simulink model "InjVlv_BlkSht"  (R2016b)
settings: configuration reference "CodeGenConfigSet" (kept outside this file)
values from neighbouring files (symbols this model uses):
  InjVlv_freqBlkShtMax_CUR = Calibration.Parameter    [init_InjVlv_BlkSht.m]    (also in init_InjVlv_BlkSht_SIL.m = Simulink.Parameter)
  InjVlv_freqBlkShtMax_CURX = Calibration.Parameter    [init_InjVlv_BlkSht.m]    (also in init_InjVlv_BlkSht_SIL.m = Simulink.Parameter)
  InjVlv_freqBlkShtMin_C = Calibration.Parameter    [init_InjVlv_BlkSht.m]    (also in init_InjVlv_BlkSht_SIL.m = Simulink.Parameter)
  InjVlv_phiBlkShtStrt_C = Calibration.Parameter    [init_InjVlv_BlkSht.m]    (also in init_InjVlv_BlkSht_SIL.m = Simulink.Parameter)
  InjVlv_phiBlkShtStrtMax_C = Calibration.Parameter    [init_InjVlv_BlkSht.m]    (also in init_InjVlv_BlkSht_SIL.m = Simulink.Parameter)
  InjVlv_phiBlkShtStrtMin_C = Calibration.Parameter    [init_InjVlv_BlkSht.m]    (also in init_InjVlv_BlkSht_SIL.m = Simulink.Parameter)
  InjVlv_swtPlausBlkShtET_C = Calibration.Parameter    [init_InjVlv_BlkSht.m]    (also in init_InjVlv_BlkSht_SIL.m = Simulink.Parameter)
  InjVlv_tiETBlkSht_MAP = Calibration.Parameter    [init_InjVlv_BlkSht.m]    (also in init_InjVlv_BlkSht_SIL.m = Simulink.Parameter)
  InjVlv_tiETBlkSht_MAPX = Calibration.Parameter    [init_InjVlv_BlkSht.m]    (also in init_InjVlv_BlkSht_SIL.m = Simulink.Parameter)
  InjVlv_tiETBlkSht_MAPY = Calibration.Parameter    [init_InjVlv_BlkSht.m]    (also in init_InjVlv_BlkSht_SIL.m = Simulink.Parameter)
  InjVlv_tiETBlkShtAft_MAP = Calibration.Parameter    [init_InjVlv_BlkSht.m]    (also in init_InjVlv_BlkSht_SIL.m = Simulink.Parameter)
  InjVlv_tiETBlkShtAft_MAPX = Calibration.Parameter    [init_InjVlv_BlkSht.m]    (also in init_InjVlv_BlkSht_SIL.m = Simulink.Parameter)
  InjVlv_tiETBlkShtAft_MAPY = Calibration.Parameter    [init_InjVlv_BlkSht.m]    (also in init_InjVlv_BlkSht_SIL.m = Simulink.Parameter)
  InjVlv_tiETBlkShtMin_C = Calibration.Parameter    [init_InjVlv_BlkSht.m]    (also in init_InjVlv_BlkSht_SIL.m = Simulink.Parameter)
  InjVlv_tiETBlkShtZFC_C = Calibration.Parameter    [init_InjVlv_BlkSht.m]    (also in init_InjVlv_BlkSht_SIL.m = Simulink.Parameter)
  SigTst_freqBlkSht_C = Calibration.Parameter    [init_InjVlv_BlkSht.m]    (also in init_InjVlv_BlkSht_SIL.m = Simulink.Parameter)
  SigTst_swtFreqBlkSht_C = Calibration.Parameter    [init_InjVlv_BlkSht.m]    (also in init_InjVlv_BlkSht_SIL.m = Simulink.Parameter)
undefined symbols (not defined in the file or in its folder): Rail_BlkShtMode_VERB, SubSysExeState_conv, Switch_conv
libraries: CXLib x1
settings Model: Creator=liangyunbo  LastModifiedBy=zhoutinglin
settings ConfigSetRef: SourceLocation=Base Workspace

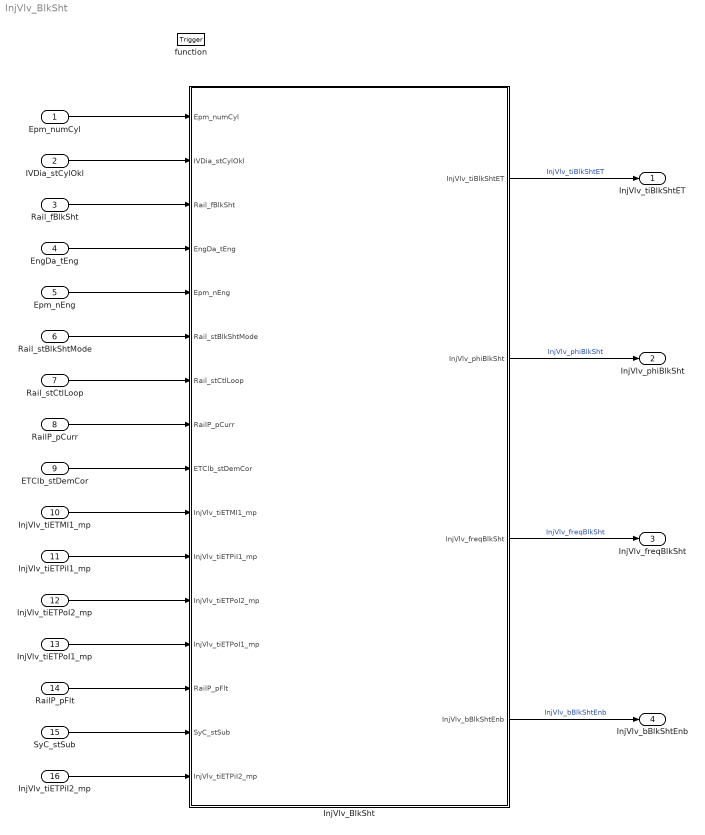
== system InjVlv_BlkSht ==
  Epm_numCyl : Inport  Description=Real number of cylinder  OutMin=0  OutMax=255  OutDataTypeStr=State_uint8
  IVDia_stCylOkl : Inport  Description=number of correct working cylinders (via bit)  Port=2  OutMin=0  OutMax=255  OutDataTypeStr=State_uint8
  Rail_fBlkSht : Inport  Tag=Hz  Description=Limited blank shot frequency  Port=3  OutMin=0  OutMax=65535  OutDataTypeStr=Freq_q1p0
  EngDa_tEng : Inport  Tag=deg  Description=Engine temperature  Port=4  OutMin=-1000  OutMax=1000  OutDataTypeStr=Temp_deg
  Epm_nEng : Inport  Tag=rpm  Description=Engine speed  Port=5  OutMin=0  OutMax=6000  OutDataTypeStr=EngSpeed_rpm
  Rail_stBlkShtMode : Inport  Description=Current active blankshot mode  Port=6  OutDataTypeStr=Enum: Rail_BlkShtMode_VERB
  Rail_stCtlLoop : Inport  Description=State of the rail pressure governor control  Port=7  OutDataTypeStr=Enum: RailCtl_State_conv
  RailP_pCurr : Inport  Tag=bar  Description=Current fuel pressure  Port=8  OutMin=0  OutMax=2500  OutDataTypeStr=RailPressure_bar
  ETClb_stDemCor : Inport  Description=Request for energizing time correction of the energizing time calibration  Port=9  OutMin=0  OutMax=255  OutDataTypeStr=State_uint8
  InjVlv_tiETMI1_mp : Inport  Tag=us  Description=Estimated MI1 energizing time  Port=10  OutMin=-13107  OutMax=13106  OutDataTypeStr=InjTime_us
  InjVlv_tiETPiI1_mp : Inport  Tag=us  Description=Estimated energizing time for PiI1  Port=11  OutMin=-13107  OutMax=13106  OutDataTypeStr=InjTime_us
  InjVlv_tiETPoI2_mp : Inport  Tag=us  Description=Start of energizing for PoI2  Port=12  OutMin=-13107  OutMax=13106  OutDataTypeStr=InjTime_us
  InjVlv_tiETPoI1_mp : Inport  Tag=us  Description=Start of energizing for PoI1  Port=13  OutMin=-13107  OutMax=13106  OutDataTypeStr=InjTime_us
  RailP_pFlt : Inport  Tag=bar  Description=Maximum rail pressure of the last 10 sampling cycle  Port=14  OutMin=0  OutMax=2500  OutDataTypeStr=RailPressure_bar
  SyC_stSub : Inport  Description=Current system/ECU sub-state  Port=15  OutDataTypeStr=Enum: SubSysExeState_conv
  InjVlv_tiETPiI2_mp : Inport  Tag=us  Description=Estimated energizing time for PiI2  Port=16  OutMin=-13107  OutMax=13106  OutDataTypeStr=InjTime_us
  function : TriggerPort  TriggerType=function-call  VariantControl=Variant
  InjVlv_BlkSht : Subsystem
  InjVlv_tiBlkShtET : Outport  Tag=us  Description=measuring points blankshot execution control / energizing time of last blakshot programmed  OutMin=-13107.2  OutMax=13106.8  OutDataTypeStr=InjTime_us
  InjVlv_phiBlkSht : Outport  Tag=CA  Description=measuring points blankshot execution control / angle of last blankshot programmed  Port=2  OutMin=-360  OutMax=0  OutDataTypeStr=Angle_CA
  InjVlv_freqBlkSht : Outport  Tag=Hz  Description=output Blank shot frequency to excute  Port=3  OutMin=0  OutMax=65535  OutDataTypeStr=Freq_q1p0
  InjVlv_bBlkShtEnb : Outport  Description=flag to indicate blank shot enable or not  Port=4  OutMin=0  OutMax=1  OutDataTypeStr=boolean
  wires:
  InjVlv_BlkSht/1(InjVlv_tiBlkShtET) -> InjVlv_tiBlkShtET/1  "InjVlv_tiBlkShtET"
  InjVlv_BlkSht/2(InjVlv_phiBlkSht) -> InjVlv_phiBlkSht/1  "InjVlv_phiBlkSht"
  InjVlv_BlkSht/3(InjVlv_freqBlkSht) -> InjVlv_freqBlkSht/1  "InjVlv_freqBlkSht"
  InjVlv_BlkSht/4(InjVlv_bBlkShtEnb) -> InjVlv_bBlkShtEnb/1  "InjVlv_bBlkShtEnb"
  ETClb_stDemCor/1 -> InjVlv_BlkSht/9(ETClb_stDemCor)
  RailP_pCurr/1 -> InjVlv_BlkSht/8(RailP_pCurr)
  Rail_stCtlLoop/1 -> InjVlv_BlkSht/7(Rail_stCtlLoop)
  Rail_stBlkShtMode/1 -> InjVlv_BlkSht/6(Rail_stBlkShtMode)
  Epm_nEng/1 -> InjVlv_BlkSht/5(Epm_nEng)
  EngDa_tEng/1 -> InjVlv_BlkSht/4(EngDa_tEng)
  Rail_fBlkSht/1 -> InjVlv_BlkSht/3(Rail_fBlkSht)
  IVDia_stCylOkl/1 -> InjVlv_BlkSht/2(IVDia_stCylOkl)
  Epm_numCyl/1 -> InjVlv_BlkSht/1(Epm_numCyl)
  InjVlv_tiETMI1_mp/1 -> InjVlv_BlkSht/10(InjVlv_tiETMI1_mp)
  InjVlv_tiETPiI1_mp/1 -> InjVlv_BlkSht/11(InjVlv_tiETPiI1_mp)
  InjVlv_tiETPoI1_mp/1 -> InjVlv_BlkSht/13(InjVlv_tiETPoI1_mp)
  InjVlv_tiETPoI2_mp/1 -> InjVlv_BlkSht/12(InjVlv_tiETPoI2_mp)
  RailP_pFlt/1 -> InjVlv_BlkSht/14(RailP_pFlt)
  SyC_stSub/1 -> InjVlv_BlkSht/15(SyC_stSub)
  InjVlv_tiETPiI2_mp/1 -> InjVlv_BlkSht/16(InjVlv_tiETPiI2_mp)

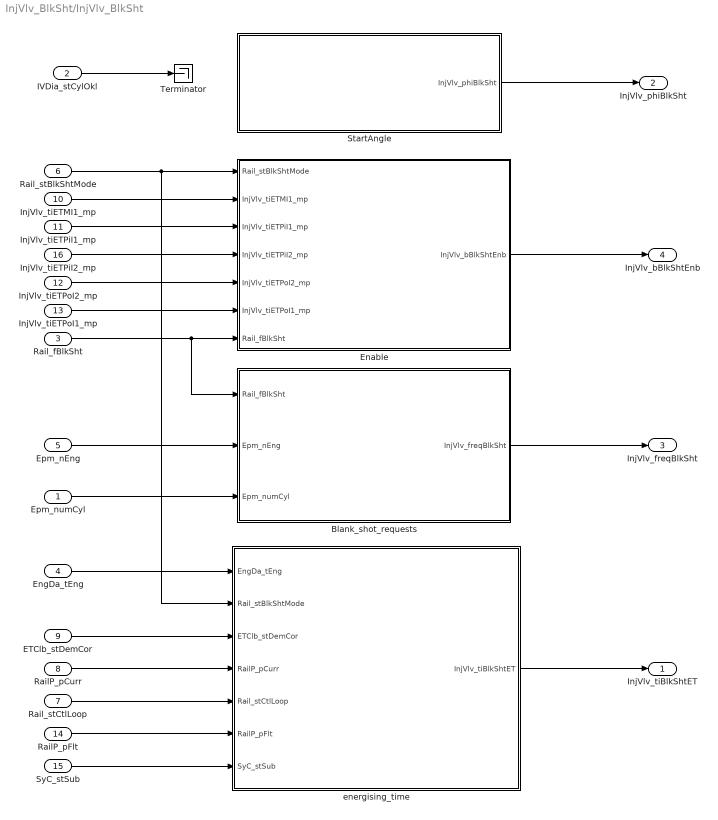
== system InjVlv_BlkSht/InjVlv_BlkSht ==
  Epm_numCyl : Inport
  IVDia_stCylOkl : Inport  Port=2
  Rail_fBlkSht : Inport  Port=3
  EngDa_tEng : Inport  Port=4
  Epm_nEng : Inport  Port=5
  Rail_stBlkShtMode : Inport  Port=6
  Rail_stCtlLoop : Inport  Port=7
  RailP_pCurr : Inport  Port=8
  ETClb_stDemCor : Inport  Port=9
  InjVlv_tiETMI1_mp : Inport  Port=10
  InjVlv_tiETPiI1_mp : Inport  Port=11
  InjVlv_tiETPoI2_mp : Inport  Port=12
  InjVlv_tiETPoI1_mp : Inport  Port=13
  RailP_pFlt : Inport  Port=14
  SyC_stSub : Inport  Port=15
  InjVlv_tiETPiI2_mp : Inport  Port=16
  Blank_shot_requests : Subsystem
  Enable : Subsystem
  StartAngle : Subsystem
  Terminator : Terminator
  energising_time : Subsystem
  InjVlv_tiBlkShtET : Outport
  InjVlv_phiBlkSht : Outport  Port=2
  InjVlv_freqBlkSht : Outport  Port=3
  InjVlv_bBlkShtEnb : Outport  Port=4
  wires:
  StartAngle/1(InjVlv_phiBlkSht) -> InjVlv_phiBlkSht/1
  Enable/1(InjVlv_bBlkShtEnb) -> InjVlv_bBlkShtEnb/1
  Rail_stBlkShtMode/1 -> Enable/1(Rail_stBlkShtMode), energising_time/2(Rail_stBlkShtMode)
  InjVlv_tiETMI1_mp/1 -> Enable/2(InjVlv_tiETMI1_mp)
  InjVlv_tiETPiI1_mp/1 -> Enable/3(InjVlv_tiETPiI1_mp)
  InjVlv_tiETPoI2_mp/1 -> Enable/5(InjVlv_tiETPoI2_mp)
  InjVlv_tiETPoI1_mp/1 -> Enable/6(InjVlv_tiETPoI1_mp)
  Blank_shot_requests/1(InjVlv_freqBlkSht) -> InjVlv_freqBlkSht/1
  energising_time/1(InjVlv_tiBlkShtET) -> InjVlv_tiBlkShtET/1
  Epm_nEng/1 -> Blank_shot_requests/2(Epm_nEng)
  EngDa_tEng/1 -> energising_time/1(EngDa_tEng)
  ETClb_stDemCor/1 -> energising_time/3(ETClb_stDemCor)
  RailP_pCurr/1 -> energising_time/4(RailP_pCurr)
  IVDia_stCylOkl/1 -> Terminator/1
  Rail_stCtlLoop/1 -> energising_time/5(Rail_stCtlLoop)
  Rail_fBlkSht/1 -> Blank_shot_requests/1(Rail_fBlkSht), Enable/7(Rail_fBlkSht)
  Epm_numCyl/1 -> Blank_shot_requests/3(Epm_numCyl)
  RailP_pFlt/1 -> energising_time/6(RailP_pFlt)
  SyC_stSub/1 -> energising_time/7(SyC_stSub)
  InjVlv_tiETPiI2_mp/1 -> Enable/4(InjVlv_tiETPiI2_mp)

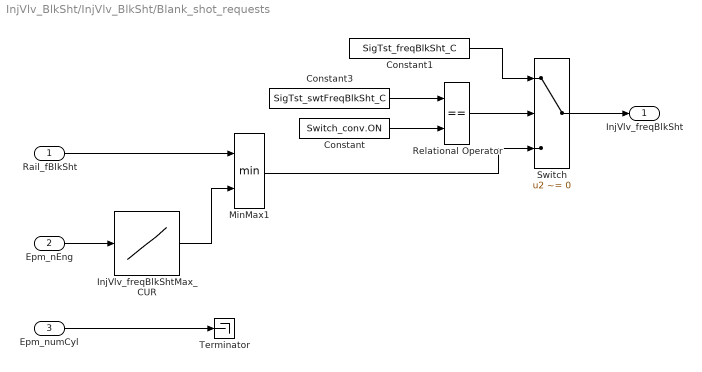
== system InjVlv_BlkSht/InjVlv_BlkSht/Blank_shot_requests ==
  Rail_fBlkSht : Inport
  Epm_nEng : Inport  Port=2
  Epm_numCyl : Inport  Port=3
  Constant : Constant  Value=Switch_conv.ON
  Constant1 : Constant  Value=SigTst_freqBlkSht_C
  Constant3 : Constant  Value=SigTst_swtFreqBlkSht_C
  InjVlv_freqBlkShtMax_CUR : Lookup_n-D  NumberOfTableDimensions=1  BreakpointsForDimension1=InjVlv_freqBlkShtMax_CURX  Table=InjVlv_freqBlkShtMax_CUR  TableDataTypeStr=Inherit: Inherit from 'Table data'  ExtrapMethod=Clip  InternalRulePriority=Speed  OutDataTypeStr=Inherit: Inherit from 'Table data'  RndMeth=Simplest
  MinMax1 : MinMax  Inputs=2  SaturateOnIntegerOverflow=on  InputSameDT=on
  Relational Operator : RelationalOperator  Operator===  OutDataTypeStr=boolean  RndMeth=Simplest
  Switch : Switch  Criteria=u2 ~= 0
  Terminator : Terminator
  InjVlv_freqBlkSht : Outport
  wires:
  Epm_nEng/1 -> InjVlv_freqBlkShtMax_CUR/1
  InjVlv_freqBlkShtMax_CUR/1 -> MinMax1/2
  Rail_fBlkSht/1 -> MinMax1/1
  Epm_numCyl/1 -> Terminator/1
  Switch/1 -> InjVlv_freqBlkSht/1
  MinMax1/1 -> Switch/3
  Relational Operator/1 -> Switch/2
  Constant/1 -> Relational Operator/2
  Constant3/1 -> Relational Operator/1
  Constant1/1 -> Switch/1

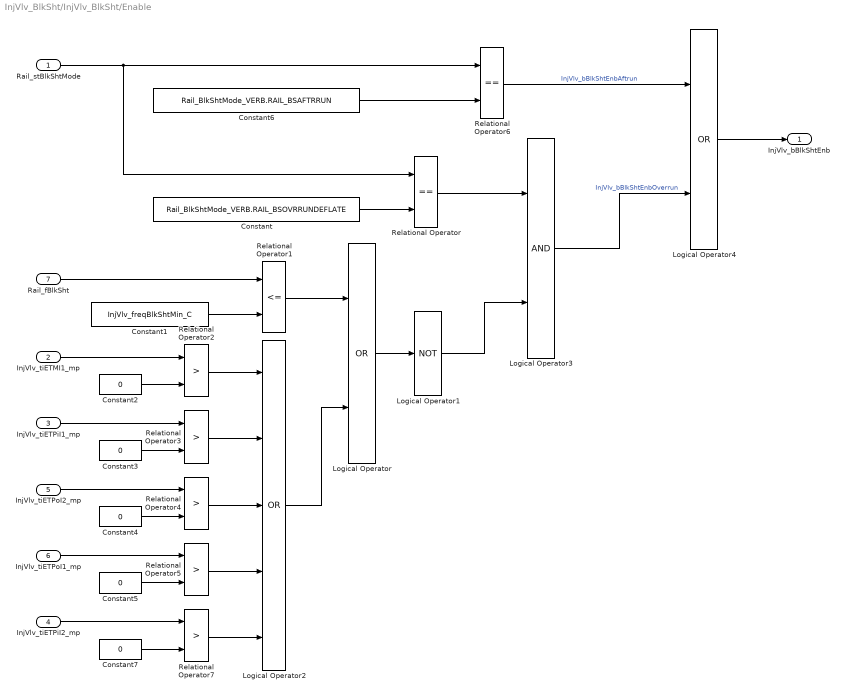
== system InjVlv_BlkSht/InjVlv_BlkSht/Enable ==
  Rail_stBlkShtMode : Inport
  InjVlv_tiETMI1_mp : Inport  Port=2
  InjVlv_tiETPiI1_mp : Inport  Port=3
  InjVlv_tiETPiI2_mp : Inport  Port=4
  InjVlv_tiETPoI2_mp : Inport  Port=5
  InjVlv_tiETPoI1_mp : Inport  Port=6
  Rail_fBlkSht : Inport  Port=7
  Constant : Constant  Value=Rail_BlkShtMode_VERB.RAIL_BSOVRRUNDEFLATE
  Constant1 : Constant  Value=InjVlv_freqBlkShtMin_C
  Constant{2..5,7} (5 alike) : Constant  Value=0  OutDataTypeStr=Inherit: Inherit via back propagation
  Constant6 : Constant  Value=Rail_BlkShtMode_VERB.RAIL_BSAFTRRUN
  Logical Operator : Logic  Operator=OR  AllPortsSameDT=off  OutDataTypeStr=boolean
  Logical Operator1 : Logic  Operator=NOT  AllPortsSameDT=off  OutDataTypeStr=boolean
  Logical Operator2 : Logic  Operator=OR  Inputs=5  AllPortsSameDT=off  OutDataTypeStr=boolean
  Logical Operator3 : Logic  AllPortsSameDT=off  OutDataTypeStr=boolean
  Logical Operator4 : Logic  Operator=OR  AllPortsSameDT=off  OutDataTypeStr=boolean
  Relational Operator : RelationalOperator  Operator===  OutDataTypeStr=boolean  RndMeth=Simplest
  Relational Operator1 : RelationalOperator  Operator=<=  OutDataTypeStr=boolean  RndMeth=Simplest
  Relational Operator{2..5,7} (5 alike) : RelationalOperator  Operator=>  OutDataTypeStr=boolean  RndMeth=Simplest  InputSameDT=on
  Relational Operator6 : RelationalOperator  Operator===  OutDataTypeStr=boolean  RndMeth=Simplest
  InjVlv_bBlkShtEnb : Outport
  wires:
  Rail_stBlkShtMode/1 -> Relational Operator/1, Relational Operator6/1
  Constant/1 -> Relational Operator/2
  Logical Operator/1 -> Logical Operator1/1
  Rail_fBlkSht/1 -> Relational Operator1/1
  Constant1/1 -> Relational Operator1/2
  InjVlv_tiETMI1_mp/1 -> Relational Operator2/1
  Constant2/1 -> Relational Operator2/2
  InjVlv_tiETPiI1_mp/1 -> Relational Operator3/1
  Constant3/1 -> Relational Operator3/2
  InjVlv_tiETPoI2_mp/1 -> Relational Operator4/1
  Constant4/1 -> Relational Operator4/2
  InjVlv_tiETPoI1_mp/1 -> Relational Operator5/1
  Constant5/1 -> Relational Operator5/2
  Relational Operator2/1 -> Logical Operator2/1
  Relational Operator3/1 -> Logical Operator2/2
  Relational Operator4/1 -> Logical Operator2/3
  Relational Operator5/1 -> Logical Operator2/4
  Relational Operator1/1 -> Logical Operator/1
  Logical Operator2/1 -> Logical Operator/2
  Relational Operator/1 -> Logical Operator3/1
  Logical Operator1/1 -> Logical Operator3/2
  Constant6/1 -> Relational Operator6/2
  Relational Operator6/1 -> Logical Operator4/1  "InjVlv_bBlkShtEnbAftrun"
  Logical Operator3/1 -> Logical Operator4/2  "InjVlv_bBlkShtEnbOverrun"
  Logical Operator4/1 -> InjVlv_bBlkShtEnb/1
  InjVlv_tiETPiI2_mp/1 -> Relational Operator7/1
  Constant7/1 -> Relational Operator7/2
  Relational Operator7/1 -> Logical Operator2/5

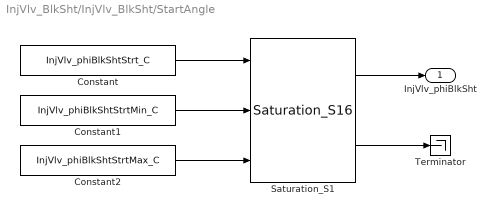
== system InjVlv_BlkSht/InjVlv_BlkSht/StartAngle ==
  Constant : Constant  Value=InjVlv_phiBlkShtStrt_C
  Constant1 : Constant  Value=InjVlv_phiBlkShtStrtMin_C
  Constant2 : Constant  Value=InjVlv_phiBlkShtStrtMax_C
  Saturation_S1 : CXLib/Saturation_S16
  Terminator : Terminator
  InjVlv_phiBlkSht : Outport
  wires:
  Saturation_S1/1 -> InjVlv_phiBlkSht/1
  Constant/1 -> Saturation_S1/1
  Constant1/1 -> Saturation_S1/2
  Constant2/1 -> Saturation_S1/3
  Saturation_S1/2 -> Terminator/1

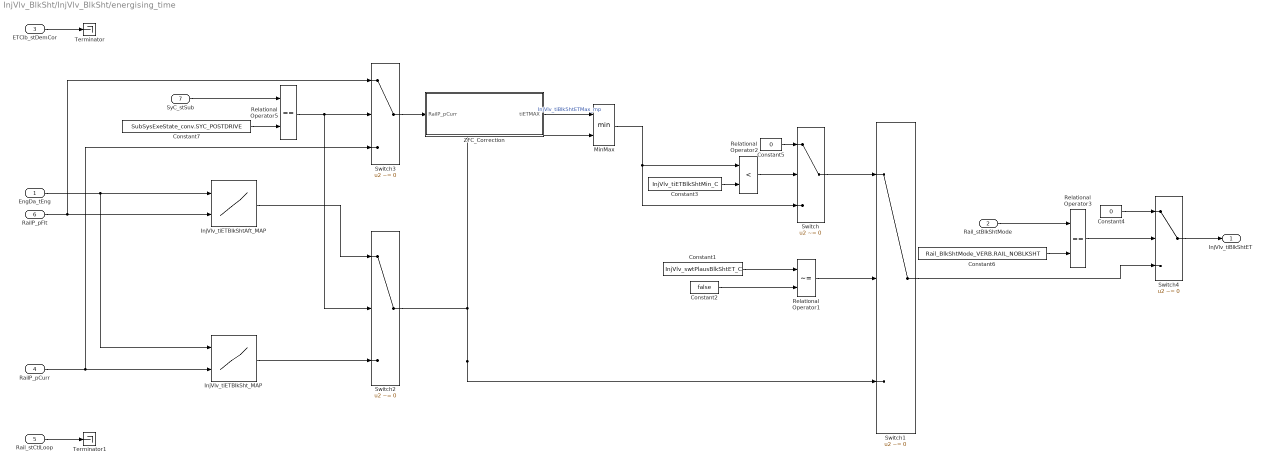
== system InjVlv_BlkSht/InjVlv_BlkSht/energising_time ==
  EngDa_tEng : Inport
  Rail_stBlkShtMode : Inport  Port=2
  ETClb_stDemCor : Inport  Port=3
  RailP_pCurr : Inport  Port=4
  Rail_stCtlLoop : Inport  Port=5
  RailP_pFlt : Inport  Port=6
  SyC_stSub : Inport  Port=7
  Constant1 : Constant  Value=InjVlv_swtPlausBlkShtET_C
  Constant2 : Constant  Value=false  OutDataTypeStr=Inherit: Inherit via back propagation
  Constant3 : Constant  Value=InjVlv_tiETBlkShtMin_C
  Constant4 : Constant  Value=0  OutDataTypeStr=Inherit: Inherit via back propagation
  Constant5 : Constant  Value=0  OutDataTypeStr=Inherit: Inherit via back propagation
  Constant6 : Constant  Value=Rail_BlkShtMode_VERB.RAIL_NOBLKSHT
  Constant7 : Constant  Value=SubSysExeState_conv.SYC_POSTDRIVE  OutDataTypeStr=Inherit: Inherit via back propagation
  InjVlv_tiETBlkShtAft_MAP : Lookup_n-D  BreakpointsForDimension1=InjVlv_tiETBlkShtAft_MAPY  BreakpointsForDimension2=InjVlv_tiETBlkShtAft_MAPX  BreakpointsForDimension1DataTypeStr=Inherit: Inherit from 'Breakpoint data'  BreakpointsForDimension2DataTypeStr=Inherit: Inherit from 'Breakpoint data'  IndexSearchMethod=Linear search  BeginIndexSearchUsingPreviousIndexResult=on  Table=InjVlv_tiETBlkShtAft_MAP  TableDataTypeStr=Inherit: Inherit from 'Table data'  ExtrapMethod=Clip  UseLastTableValue=on  InternalRulePriority=Speed  OutDataTypeStr=Inherit: Inherit from 'Table data'  RndMeth=Simplest  SaturateOnIntegerOverflow=on
  InjVlv_tiETBlkSht_MAP : Lookup_n-D  BreakpointsForDimension1=InjVlv_tiETBlkSht_MAPY  BreakpointsForDimension2=InjVlv_tiETBlkSht_MAPX  BreakpointsForDimension1DataTypeStr=Inherit: Inherit from 'Breakpoint data'  BreakpointsForDimension2DataTypeStr=Inherit: Inherit from 'Breakpoint data'  IndexSearchMethod=Linear search  BeginIndexSearchUsingPreviousIndexResult=on  Table=InjVlv_tiETBlkSht_MAP  TableDataTypeStr=Inherit: Inherit from 'Table data'  ExtrapMethod=Clip  UseLastTableValue=on  InternalRulePriority=Speed  OutDataTypeStr=Inherit: Inherit from 'Table data'  RndMeth=Simplest  SaturateOnIntegerOverflow=on
  MinMax : MinMax  Inputs=2  SaturateOnIntegerOverflow=on  InputSameDT=on
  Relational Operator1 : RelationalOperator  Operator=~=  OutDataTypeStr=boolean  RndMeth=Simplest  InputSameDT=on
  Relational Operator2 : RelationalOperator  Operator=<  OutDataTypeStr=boolean  RndMeth=Simplest  InputSameDT=on
  Relational Operator3 : RelationalOperator  Operator===  OutDataTypeStr=boolean  RndMeth=Simplest  InputSameDT=on
  Relational Operator5 : RelationalOperator  Operator===  OutDataTypeStr=boolean  RndMeth=Simplest  InputSameDT=on
  Switch : Switch  Criteria=u2 ~= 0  SaturateOnIntegerOverflow=on  InputSameDT=on
  Switch1 : Switch  Criteria=u2 ~= 0  SaturateOnIntegerOverflow=on  InputSameDT=on
  Switch2 : Switch  Criteria=u2 ~= 0
  Switch3 : Switch  Criteria=u2 ~= 0
  Switch4 : Switch  Criteria=u2 ~= 0  SaturateOnIntegerOverflow=on  InputSameDT=on
  Terminator : Terminator
  Terminator1 : Terminator
  ZFC_Correction : Subsystem
  InjVlv_tiBlkShtET : Outport
  wires:
  Constant1/1 -> Relational Operator1/1
  Switch/1 -> Switch1/1
  Constant5/1 -> Switch/1
  Constant3/1 -> Relational Operator2/2
  Constant2/1 -> Relational Operator1/2
  Relational Operator2/1 -> Switch/2
  EngDa_tEng/1 -> InjVlv_tiETBlkSht_MAP/1, InjVlv_tiETBlkShtAft_MAP/1
  Relational Operator1/1 -> Switch1/2
  ZFC_Correction/1(tiETMAX) -> MinMax/1  "InjVlv_tiBlkShtETMax_mp"
  MinMax/1 -> Switch/3, Relational Operator2/1
  ETClb_stDemCor/1 -> Terminator/1
  RailP_pFlt/1 -> Switch3/1, InjVlv_tiETBlkShtAft_MAP/2
  Constant7/1 -> Relational Operator5/2
  SyC_stSub/1 -> Relational Operator5/1
  Relational Operator5/1 -> Switch2/2, Switch3/2
  InjVlv_tiETBlkSht_MAP/1 -> Switch2/3
  InjVlv_tiETBlkShtAft_MAP/1 -> Switch2/1
  RailP_pCurr/1 -> Switch3/3, InjVlv_tiETBlkSht_MAP/2
  Switch3/1 -> ZFC_Correction/1(RailP_pCurr)
  Switch2/1 -> MinMax/2, Switch1/3
  Rail_stCtlLoop/1 -> Terminator1/1
  Switch4/1 -> InjVlv_tiBlkShtET/1
  Rail_stBlkShtMode/1 -> Relational Operator3/1
  Constant6/1 -> Relational Operator3/2
  Relational Operator3/1 -> Switch4/2
  Constant4/1 -> Switch4/1
  Switch1/1 -> Switch4/3

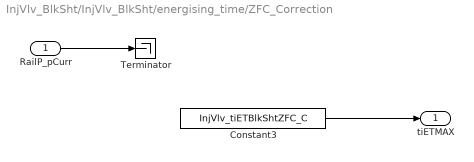
== system InjVlv_BlkSht/InjVlv_BlkSht/energising_time/ZFC_Correction ==
  RailP_pCurr : Inport
  Constant3 : Constant  Value=InjVlv_tiETBlkShtZFC_C
  Terminator : Terminator
  tiETMAX : Outport
  wires:
  RailP_pCurr/1 -> Terminator/1
  Constant3/1 -> tiETMAX/1
